simulink model "Lab2"  (R2024b)
settings: Solver=FixedStepAuto  StartTime=0.0  StopTime=10.0  RelTol=1e-3  EnableMultiTasking=on
undefined symbols (not defined in the file): BOOL, DINT, OTL, slplc
libraries: simulink x8, arduinolib x3
(part 2 of 8)

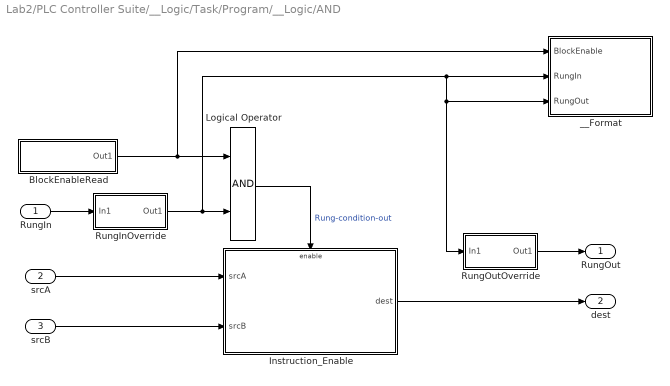
== system Lab2/PLC Controller Suite/__Logic/Task/Program/__Logic/AND ==
  RungIn : Inport  OutDataTypeStr=BOOL  PortDimensions=1
  srcA : Inport  Port=2  PortDimensions=1
  srcB : Inport  Port=3  PortDimensions=1
  BlockEnableRead : Subsystem  DisableCoverage=on  TreatAsAtomicUnit=on  mask{PLCLabelTag=_Block_Enable, PLCBlockType=BlockEnableRead}
      mask prompts: PLCLabelTag "Label Tag:"
      mask init:
      | block = gcb;
      | maskObj = Simulink.Mask.get(block);
      | maskObj.Display = sprintf('disp(''%s'');', PLCLabelTag);
      mask Help: web([docroot '/plccoder/ref/blockenableread' '.html']);
      mask DialogControl PLCBlockTitle Prompt: Block Enable Read
      mask Display: disp('_Block_Enable');
  Instruction_Enable : Subsystem  TreatAsAtomicUnit=on
  Logical Operator : Logic  OutDataTypeStr=BOOL
  RungInOverride : Subsystem  DisableCoverage=on  TreatAsAtomicUnit=on
  RungOutOverride : Subsystem  DisableCoverage=on  TreatAsAtomicUnit=on
  __Format : MATLAB Function  Tag=PLC_Format_FC  Priority=20  DisableCoverage=on  InitFcn=slplc.utils.setBlockAppearance('reset');  StopFcn=slplc.utils.setBlockAppearance('reset');  TreatAsAtomicUnit=on
  RungOut : Outport  OutDataTypeStr=BOOL  PortDimensions=1  VectorParamsAs1DForOutWhenUnconnected=off
  dest : Outport  Port=2  PortDimensions=1  VectorParamsAs1DForOutWhenUnconnected=off
  wires:
  RungOutOverride/1(Out1) -> RungOut/1
  RungIn/1 -> RungInOverride/1(In1)
  BlockEnableRead/1(Out1) -> Logical Operator/1, __Format/1(BlockEnable)
  srcB/1 -> Instruction_Enable/2(srcB)
  RungInOverride/1(Out1) -> Logical Operator/2, RungOutOverride/1(In1), __Format/3(RungOut), __Format/2(RungIn)
  Instruction_Enable/1(dest) -> dest/1
  srcA/1 -> Instruction_Enable/1(srcA)
  Logical Operator/1 -> Instruction_Enable/Enable  "Rung-condition-out"

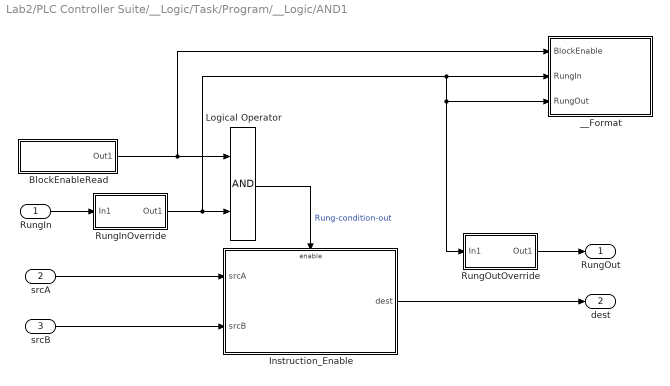
== system Lab2/PLC Controller Suite/__Logic/Task/Program/__Logic/AND1 ==
  RungIn : Inport  OutDataTypeStr=BOOL  PortDimensions=1
  srcA : Inport  Port=2  PortDimensions=1
  srcB : Inport  Port=3  PortDimensions=1
  BlockEnableRead : Subsystem  DisableCoverage=on  TreatAsAtomicUnit=on  mask{PLCLabelTag=_Block_Enable, PLCBlockType=BlockEnableRead}
      mask prompts: PLCLabelTag "Label Tag:"
      mask init:
      | block = gcb;
      | maskObj = Simulink.Mask.get(block);
      | maskObj.Display = sprintf('disp(''%s'');', PLCLabelTag);
      mask Help: web([docroot '/plccoder/ref/blockenableread' '.html']);
      mask DialogControl PLCBlockTitle Prompt: Block Enable Read
      mask Display: disp('_Block_Enable');
  Instruction_Enable : Subsystem  TreatAsAtomicUnit=on
  Logical Operator : Logic  OutDataTypeStr=BOOL
  RungInOverride : Subsystem  DisableCoverage=on  TreatAsAtomicUnit=on
  RungOutOverride : Subsystem  DisableCoverage=on  TreatAsAtomicUnit=on
  __Format : MATLAB Function  Tag=PLC_Format_FC  Priority=20  DisableCoverage=on  InitFcn=slplc.utils.setBlockAppearance('reset');  StopFcn=slplc.utils.setBlockAppearance('reset');  TreatAsAtomicUnit=on
  RungOut : Outport  OutDataTypeStr=BOOL  PortDimensions=1  VectorParamsAs1DForOutWhenUnconnected=off
  dest : Outport  Port=2  PortDimensions=1  VectorParamsAs1DForOutWhenUnconnected=off
  wires:
  RungOutOverride/1(Out1) -> RungOut/1
  RungIn/1 -> RungInOverride/1(In1)
  BlockEnableRead/1(Out1) -> Logical Operator/1, __Format/1(BlockEnable)
  srcB/1 -> Instruction_Enable/2(srcB)
  RungInOverride/1(Out1) -> Logical Operator/2, RungOutOverride/1(In1), __Format/3(RungOut), __Format/2(RungIn)
  Instruction_Enable/1(dest) -> dest/1
  srcA/1 -> Instruction_Enable/1(srcA)
  Logical Operator/1 -> Instruction_Enable/Enable  "Rung-condition-out"

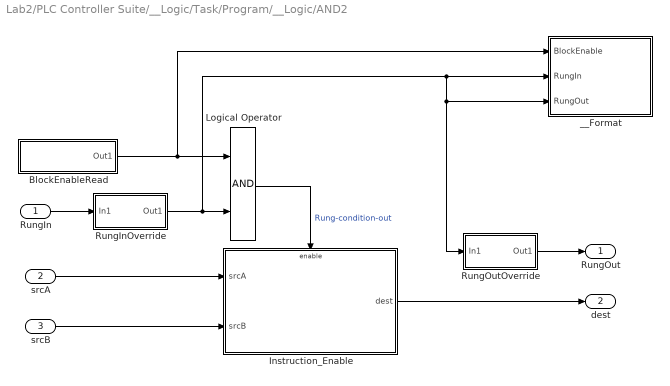
== system Lab2/PLC Controller Suite/__Logic/Task/Program/__Logic/AND2 ==
  RungIn : Inport  OutDataTypeStr=BOOL  PortDimensions=1
  srcA : Inport  Port=2  PortDimensions=1
  srcB : Inport  Port=3  PortDimensions=1
  BlockEnableRead : Subsystem  DisableCoverage=on  TreatAsAtomicUnit=on  mask{PLCLabelTag=_Block_Enable, PLCBlockType=BlockEnableRead}
      mask prompts: PLCLabelTag "Label Tag:"
      mask init:
      | block = gcb;
      | maskObj = Simulink.Mask.get(block);
      | maskObj.Display = sprintf('disp(''%s'');', PLCLabelTag);
      mask Help: web([docroot '/plccoder/ref/blockenableread' '.html']);
      mask DialogControl PLCBlockTitle Prompt: Block Enable Read
      mask Display: disp('_Block_Enable');
  Instruction_Enable : Subsystem  TreatAsAtomicUnit=on
  Logical Operator : Logic  OutDataTypeStr=BOOL
  RungInOverride : Subsystem  DisableCoverage=on  TreatAsAtomicUnit=on
  RungOutOverride : Subsystem  DisableCoverage=on  TreatAsAtomicUnit=on
  __Format : MATLAB Function  Tag=PLC_Format_FC  Priority=20  DisableCoverage=on  InitFcn=slplc.utils.setBlockAppearance('reset');  StopFcn=slplc.utils.setBlockAppearance('reset');  TreatAsAtomicUnit=on
  RungOut : Outport  OutDataTypeStr=BOOL  PortDimensions=1  VectorParamsAs1DForOutWhenUnconnected=off
  dest : Outport  Port=2  PortDimensions=1  VectorParamsAs1DForOutWhenUnconnected=off
  wires:
  RungOutOverride/1(Out1) -> RungOut/1
  RungIn/1 -> RungInOverride/1(In1)
  BlockEnableRead/1(Out1) -> Logical Operator/1, __Format/1(BlockEnable)
  srcB/1 -> Instruction_Enable/2(srcB)
  RungInOverride/1(Out1) -> Logical Operator/2, RungOutOverride/1(In1), __Format/3(RungOut), __Format/2(RungIn)
  Instruction_Enable/1(dest) -> dest/1
  srcA/1 -> Instruction_Enable/1(srcA)
  Logical Operator/1 -> Instruction_Enable/Enable  "Rung-condition-out"

== system Lab2/PLC Controller Suite/__Logic/Task/Program/__Logic/Add Rungs ==

== system Lab2/PLC Controller Suite/__Logic/Task/Program/__Logic/Add Single Rung ==

== system Lab2/PLC Controller Suite/__Logic/Task/Program/__Logic/Junction ==
  RungIn1 : Inport
  RungIn2 : Inport  Port=2
  BlockEnableRead : Subsystem  DisableCoverage=on  TreatAsAtomicUnit=on  mask{PLCLabelTag=_Block_Enable, PLCBlockType=BlockEnableRead}
      mask prompts: PLCLabelTag "Label Tag:"
      mask init:
      | block = gcb;
      | maskObj = Simulink.Mask.get(block);
      | maskObj.Display = sprintf('disp(''%s'');', PLCLabelTag);
      mask Help: web([docroot '/plccoder/ref/blockenableread' '.html']);
      mask DialogControl PLCBlockTitle Prompt: Block Enable Read
      mask Display: disp('_Block_Enable');
  __Enable : Subsystem  TreatAsAtomicUnit=on
  __Format : MATLAB Function  Tag=PLC_Format_Joint  Priority=20  DisableCoverage=on  InitFcn=slplc.utils.setBlockAppearance('reset', '', {'black', 'black'});  StopFcn=slplc.utils.setBlockAppearance('reset', '', {'black', 'black'});  TreatAsAtomicUnit=on
  RungOut : Outport  VectorParamsAs1DForOutWhenUnconnected=off
  wires:
  __Enable/1(RungOut) -> RungOut/1, __Format/2(RungOut)
  RungIn2/1 -> __Enable/2(RungIn2)
  RungIn1/1 -> __Enable/1(RungIn1)
  BlockEnableRead/1(Out1) -> __Enable/Enable, __Format/1(BlockEnable)

== system Lab2/PLC Controller Suite/__Logic/Task/Program/__Logic/Junction1 ==
  RungIn1 : Inport
  RungIn2 : Inport  Port=2
  BlockEnableRead : Subsystem  DisableCoverage=on  TreatAsAtomicUnit=on  mask{PLCLabelTag=_Block_Enable, PLCBlockType=BlockEnableRead}
      mask prompts: PLCLabelTag "Label Tag:"
      mask init:
      | block = gcb;
      | maskObj = Simulink.Mask.get(block);
      | maskObj.Display = sprintf('disp(''%s'');', PLCLabelTag);
      mask Help: web([docroot '/plccoder/ref/blockenableread' '.html']);
      mask DialogControl PLCBlockTitle Prompt: Block Enable Read
      mask Display: disp('_Block_Enable');
  __Enable : Subsystem  TreatAsAtomicUnit=on
  __Format : MATLAB Function  Tag=PLC_Format_Joint  Priority=20  DisableCoverage=on  InitFcn=slplc.utils.setBlockAppearance('reset', '', {'black', 'black'});  StopFcn=slplc.utils.setBlockAppearance('reset', '', {'black', 'black'});  TreatAsAtomicUnit=on
  RungOut : Outport  VectorParamsAs1DForOutWhenUnconnected=off
  wires:
  __Enable/1(RungOut) -> RungOut/1, __Format/2(RungOut)
  RungIn2/1 -> __Enable/2(RungIn2)
  RungIn1/1 -> __Enable/1(RungIn1)
  BlockEnableRead/1(Out1) -> __Enable/Enable, __Format/1(BlockEnable)

== system Lab2/PLC Controller Suite/__Logic/Task/Program/__Logic/Junction2 ==
  RungIn1 : Inport
  RungIn2 : Inport  Port=2
  BlockEnableRead : Subsystem  DisableCoverage=on  TreatAsAtomicUnit=on  mask{PLCLabelTag=_Block_Enable, PLCBlockType=BlockEnableRead}
      mask prompts: PLCLabelTag "Label Tag:"
      mask init:
      | block = gcb;
      | maskObj = Simulink.Mask.get(block);
      | maskObj.Display = sprintf('disp(''%s'');', PLCLabelTag);
      mask Help: web([docroot '/plccoder/ref/blockenableread' '.html']);
      mask DialogControl PLCBlockTitle Prompt: Block Enable Read
      mask Display: disp('_Block_Enable');
  __Enable : Subsystem  TreatAsAtomicUnit=on
  __Format : MATLAB Function  Tag=PLC_Format_Joint  Priority=20  DisableCoverage=on  InitFcn=slplc.utils.setBlockAppearance('reset', '', {'black', 'black'});  StopFcn=slplc.utils.setBlockAppearance('reset', '', {'black', 'black'});  TreatAsAtomicUnit=on
  RungOut : Outport  VectorParamsAs1DForOutWhenUnconnected=off
  wires:
  __Enable/1(RungOut) -> RungOut/1, __Format/2(RungOut)
  RungIn2/1 -> __Enable/2(RungIn2)
  RungIn1/1 -> __Enable/1(RungIn1)
  BlockEnableRead/1(Out1) -> __Enable/Enable, __Format/1(BlockEnable)

== system Lab2/PLC Controller Suite/__Logic/Task/Program/__Logic/Junction3 ==
  RungIn1 : Inport
  RungIn2 : Inport  Port=2
  BlockEnableRead : Subsystem  DisableCoverage=on  TreatAsAtomicUnit=on  mask{PLCLabelTag=_Block_Enable, PLCBlockType=BlockEnableRead}
      mask prompts: PLCLabelTag "Label Tag:"
      mask init:
      | block = gcb;
      | maskObj = Simulink.Mask.get(block);
      | maskObj.Display = sprintf('disp(''%s'');', PLCLabelTag);
      mask Help: web([docroot '/plccoder/ref/blockenableread' '.html']);
      mask DialogControl PLCBlockTitle Prompt: Block Enable Read
      mask Display: disp('_Block_Enable');
  __Enable : Subsystem  TreatAsAtomicUnit=on
  __Format : MATLAB Function  Tag=PLC_Format_Joint  Priority=20  DisableCoverage=on  InitFcn=slplc.utils.setBlockAppearance('reset', '', {'black', 'black'});  StopFcn=slplc.utils.setBlockAppearance('reset', '', {'black', 'black'});  TreatAsAtomicUnit=on
  RungOut : Outport  VectorParamsAs1DForOutWhenUnconnected=off
  wires:
  __Enable/1(RungOut) -> RungOut/1, __Format/2(RungOut)
  RungIn2/1 -> __Enable/2(RungIn2)
  RungIn1/1 -> __Enable/1(RungIn1)
  BlockEnableRead/1(Out1) -> __Enable/Enable, __Format/1(BlockEnable)

== system Lab2/PLC Controller Suite/__Logic/Task/Program/__Logic/Junction4 ==
  RungIn1 : Inport
  RungIn2 : Inport  Port=2
  BlockEnableRead : Subsystem  DisableCoverage=on  TreatAsAtomicUnit=on  mask{PLCLabelTag=_Block_Enable, PLCBlockType=BlockEnableRead}
      mask prompts: PLCLabelTag "Label Tag:"
      mask init:
      | block = gcb;
      | maskObj = Simulink.Mask.get(block);
      | maskObj.Display = sprintf('disp(''%s'');', PLCLabelTag);
      mask Help: web([docroot '/plccoder/ref/blockenableread' '.html']);
      mask DialogControl PLCBlockTitle Prompt: Block Enable Read
      mask Display: disp('_Block_Enable');
  __Enable : Subsystem  TreatAsAtomicUnit=on
  __Format : MATLAB Function  Tag=PLC_Format_Joint  Priority=20  DisableCoverage=on  InitFcn=slplc.utils.setBlockAppearance('reset', '', {'black', 'black'});  StopFcn=slplc.utils.setBlockAppearance('reset', '', {'black', 'black'});  TreatAsAtomicUnit=on
  RungOut : Outport  VectorParamsAs1DForOutWhenUnconnected=off
  wires:
  __Enable/1(RungOut) -> RungOut/1, __Format/2(RungOut)
  RungIn2/1 -> __Enable/2(RungIn2)
  RungIn1/1 -> __Enable/1(RungIn1)
  BlockEnableRead/1(Out1) -> __Enable/Enable, __Format/1(BlockEnable)

== system Lab2/PLC Controller Suite/__Logic/Task/Program/__Logic/LES ==
  RungIn : Inport  OutDataTypeStr=BOOL  PortDimensions=1
  srcA : Inport  Port=2  PortDimensions=1
  srcB : Inport  Port=3  PortDimensions=1
  BlockEnableRead : Subsystem  DisableCoverage=on  TreatAsAtomicUnit=on  mask{PLCLabelTag=_Block_Enable, PLCBlockType=BlockEnableRead}
      mask prompts: PLCLabelTag "Label Tag:"
      mask init:
      | block = gcb;
      | maskObj = Simulink.Mask.get(block);
      | maskObj.Display = sprintf('disp(''%s'');', PLCLabelTag);
      mask Help: web([docroot '/plccoder/ref/blockenableread' '.html']);
      mask DialogControl PLCBlockTitle Prompt: Block Enable Read
      mask Display: disp('_Block_Enable');
  Instruction_Enable : Subsystem  TreatAsAtomicUnit=on
  RungInOverride : Subsystem  DisableCoverage=on  TreatAsAtomicUnit=on
  __Format : MATLAB Function  Tag=PLC_Format_FC  Priority=20  DisableCoverage=on  InitFcn=slplc.utils.setBlockAppearance('reset');  StopFcn=slplc.utils.setBlockAppearance('reset');  TreatAsAtomicUnit=on
  RungOut : Outport  OutDataTypeStr=BOOL  PortDimensions=1  VectorParamsAs1DForOutWhenUnconnected=off
  wires:
  RungIn/1 -> RungInOverride/1(In1)
  srcB/1 -> Instruction_Enable/3(srcB)
  Instruction_Enable/1(Rung-condition-out) -> RungOut/1, __Format/3(RungOut)
  BlockEnableRead/1(Out1) -> Instruction_Enable/Enable, __Format/1(BlockEnable)
  RungInOverride/1(Out1) -> Instruction_Enable/1(Rung-condition-in), __Format/2(RungIn)
  srcA/1 -> Instruction_Enable/2(srcA)

== system Lab2/PLC Controller Suite/__Logic/Task/Program/__Logic/LES1 ==
  RungIn : Inport  OutDataTypeStr=BOOL  PortDimensions=1
  srcA : Inport  Port=2  PortDimensions=1
  srcB : Inport  Port=3  PortDimensions=1
  BlockEnableRead : Subsystem  DisableCoverage=on  TreatAsAtomicUnit=on  mask{PLCLabelTag=_Block_Enable, PLCBlockType=BlockEnableRead}
      mask prompts: PLCLabelTag "Label Tag:"
      mask init:
      | block = gcb;
      | maskObj = Simulink.Mask.get(block);
      | maskObj.Display = sprintf('disp(''%s'');', PLCLabelTag);
      mask Help: web([docroot '/plccoder/ref/blockenableread' '.html']);
      mask DialogControl PLCBlockTitle Prompt: Block Enable Read
      mask Display: disp('_Block_Enable');
  Instruction_Enable : Subsystem  TreatAsAtomicUnit=on
  RungInOverride : Subsystem  DisableCoverage=on  TreatAsAtomicUnit=on
  __Format : MATLAB Function  Tag=PLC_Format_FC  Priority=20  DisableCoverage=on  InitFcn=slplc.utils.setBlockAppearance('reset');  StopFcn=slplc.utils.setBlockAppearance('reset');  TreatAsAtomicUnit=on
  RungOut : Outport  OutDataTypeStr=BOOL  PortDimensions=1  VectorParamsAs1DForOutWhenUnconnected=off
  wires:
  RungIn/1 -> RungInOverride/1(In1)
  srcB/1 -> Instruction_Enable/3(srcB)
  Instruction_Enable/1(Rung-condition-out) -> RungOut/1, __Format/3(RungOut)
  BlockEnableRead/1(Out1) -> Instruction_Enable/Enable, __Format/1(BlockEnable)
  RungInOverride/1(Out1) -> Instruction_Enable/1(Rung-condition-in), __Format/2(RungIn)
  srcA/1 -> Instruction_Enable/2(srcA)

== system Lab2/PLC Controller Suite/__Logic/Task/Program/__Logic/LES2 ==
  RungIn : Inport  OutDataTypeStr=BOOL  PortDimensions=1
  srcA : Inport  Port=2  PortDimensions=1
  srcB : Inport  Port=3  PortDimensions=1
  BlockEnableRead : Subsystem  DisableCoverage=on  TreatAsAtomicUnit=on  mask{PLCLabelTag=_Block_Enable, PLCBlockType=BlockEnableRead}
      mask prompts: PLCLabelTag "Label Tag:"
      mask init:
      | block = gcb;
      | maskObj = Simulink.Mask.get(block);
      | maskObj.Display = sprintf('disp(''%s'');', PLCLabelTag);
      mask Help: web([docroot '/plccoder/ref/blockenableread' '.html']);
      mask DialogControl PLCBlockTitle Prompt: Block Enable Read
      mask Display: disp('_Block_Enable');
  Instruction_Enable : Subsystem  TreatAsAtomicUnit=on
  RungInOverride : Subsystem  DisableCoverage=on  TreatAsAtomicUnit=on
  __Format : MATLAB Function  Tag=PLC_Format_FC  Priority=20  DisableCoverage=on  InitFcn=slplc.utils.setBlockAppearance('reset');  StopFcn=slplc.utils.setBlockAppearance('reset');  TreatAsAtomicUnit=on
  RungOut : Outport  OutDataTypeStr=BOOL  PortDimensions=1  VectorParamsAs1DForOutWhenUnconnected=off
  wires:
  RungIn/1 -> RungInOverride/1(In1)
  srcB/1 -> Instruction_Enable/3(srcB)
  Instruction_Enable/1(Rung-condition-out) -> RungOut/1, __Format/3(RungOut)
  BlockEnableRead/1(Out1) -> Instruction_Enable/Enable, __Format/1(BlockEnable)
  RungInOverride/1(Out1) -> Instruction_Enable/1(Rung-condition-in), __Format/2(RungIn)
  srcA/1 -> Instruction_Enable/2(srcA)

== system Lab2/PLC Controller Suite/__Logic/Task/Program/__Logic/LES3 ==
  RungIn : Inport  OutDataTypeStr=BOOL  PortDimensions=1
  srcA : Inport  Port=2  PortDimensions=1
  srcB : Inport  Port=3  PortDimensions=1
  BlockEnableRead : Subsystem  DisableCoverage=on  TreatAsAtomicUnit=on  mask{PLCLabelTag=_Block_Enable, PLCBlockType=BlockEnableRead}
      mask prompts: PLCLabelTag "Label Tag:"
      mask init:
      | block = gcb;
      | maskObj = Simulink.Mask.get(block);
      | maskObj.Display = sprintf('disp(''%s'');', PLCLabelTag);
      mask Help: web([docroot '/plccoder/ref/blockenableread' '.html']);
      mask DialogControl PLCBlockTitle Prompt: Block Enable Read
      mask Display: disp('_Block_Enable');
  Instruction_Enable : Subsystem  TreatAsAtomicUnit=on
  RungInOverride : Subsystem  DisableCoverage=on  TreatAsAtomicUnit=on
  __Format : MATLAB Function  Tag=PLC_Format_FC  Priority=20  DisableCoverage=on  InitFcn=slplc.utils.setBlockAppearance('reset');  StopFcn=slplc.utils.setBlockAppearance('reset');  TreatAsAtomicUnit=on
  RungOut : Outport  OutDataTypeStr=BOOL  PortDimensions=1  VectorParamsAs1DForOutWhenUnconnected=off
  wires:
  RungIn/1 -> RungInOverride/1(In1)
  srcB/1 -> Instruction_Enable/3(srcB)
  Instruction_Enable/1(Rung-condition-out) -> RungOut/1, __Format/3(RungOut)
  BlockEnableRead/1(Out1) -> Instruction_Enable/Enable, __Format/1(BlockEnable)
  RungInOverride/1(Out1) -> Instruction_Enable/1(Rung-condition-in), __Format/2(RungIn)
  srcA/1 -> Instruction_Enable/2(srcA)

== system Lab2/PLC Controller Suite/__Logic/Task/Program/__Logic/LES4 ==
  RungIn : Inport  OutDataTypeStr=BOOL  PortDimensions=1
  srcA : Inport  Port=2  PortDimensions=1
  srcB : Inport  Port=3  PortDimensions=1
  BlockEnableRead : Subsystem  DisableCoverage=on  TreatAsAtomicUnit=on  mask{PLCLabelTag=_Block_Enable, PLCBlockType=BlockEnableRead}
      mask prompts: PLCLabelTag "Label Tag:"
      mask init:
      | block = gcb;
      | maskObj = Simulink.Mask.get(block);
      | maskObj.Display = sprintf('disp(''%s'');', PLCLabelTag);
      mask Help: web([docroot '/plccoder/ref/blockenableread' '.html']);
      mask DialogControl PLCBlockTitle Prompt: Block Enable Read
      mask Display: disp('_Block_Enable');
  Instruction_Enable : Subsystem  TreatAsAtomicUnit=on
  RungInOverride : Subsystem  DisableCoverage=on  TreatAsAtomicUnit=on
  __Format : MATLAB Function  Tag=PLC_Format_FC  Priority=20  DisableCoverage=on  InitFcn=slplc.utils.setBlockAppearance('reset');  StopFcn=slplc.utils.setBlockAppearance('reset');  TreatAsAtomicUnit=on
  RungOut : Outport  OutDataTypeStr=BOOL  PortDimensions=1  VectorParamsAs1DForOutWhenUnconnected=off
  wires:
  RungIn/1 -> RungInOverride/1(In1)
  srcB/1 -> Instruction_Enable/3(srcB)
  Instruction_Enable/1(Rung-condition-out) -> RungOut/1, __Format/3(RungOut)
  BlockEnableRead/1(Out1) -> Instruction_Enable/Enable, __Format/1(BlockEnable)
  RungInOverride/1(Out1) -> Instruction_Enable/1(Rung-condition-in), __Format/2(RungIn)
  srcA/1 -> Instruction_Enable/2(srcA)

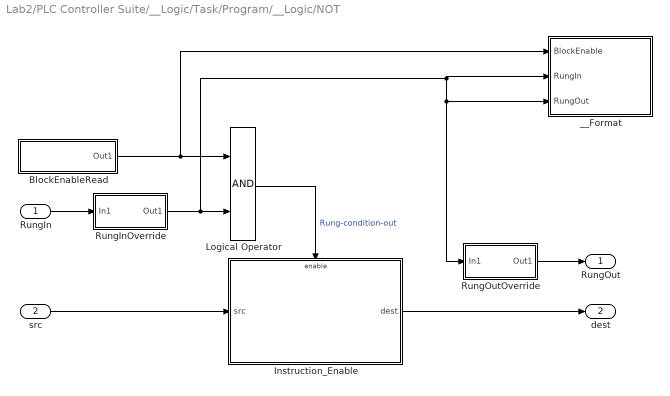
== system Lab2/PLC Controller Suite/__Logic/Task/Program/__Logic/NOT ==
  RungIn : Inport  OutDataTypeStr=BOOL  PortDimensions=1
  src : Inport  Port=2  PortDimensions=1
  BlockEnableRead : Subsystem  DisableCoverage=on  TreatAsAtomicUnit=on  mask{PLCLabelTag=_Block_Enable, PLCBlockType=BlockEnableRead}
      mask prompts: PLCLabelTag "Label Tag:"
      mask init:
      | block = gcb;
      | maskObj = Simulink.Mask.get(block);
      | maskObj.Display = sprintf('disp(''%s'');', PLCLabelTag);
      mask Help: web([docroot '/plccoder/ref/blockenableread' '.html']);
      mask DialogControl PLCBlockTitle Prompt: Block Enable Read
      mask Display: disp('_Block_Enable');
  Instruction_Enable : Subsystem  TreatAsAtomicUnit=on
  Logical Operator : Logic  OutDataTypeStr=BOOL
  RungInOverride : Subsystem  DisableCoverage=on  TreatAsAtomicUnit=on
  RungOutOverride : Subsystem  DisableCoverage=on  TreatAsAtomicUnit=on
  __Format : MATLAB Function  Tag=PLC_Format_FC  Priority=20  DisableCoverage=on  InitFcn=slplc.utils.setBlockAppearance('reset');  StopFcn=slplc.utils.setBlockAppearance('reset');  TreatAsAtomicUnit=on
  RungOut : Outport  OutDataTypeStr=BOOL  PortDimensions=1  VectorParamsAs1DForOutWhenUnconnected=off
  dest : Outport  Port=2  PortDimensions=1  VectorParamsAs1DForOutWhenUnconnected=off
  wires:
  BlockEnableRead/1(Out1) -> Logical Operator/1, __Format/1(BlockEnable)
  RungInOverride/1(Out1) -> RungOutOverride/1(In1), __Format/3(RungOut), __Format/2(RungIn), Logical Operator/2
  RungOutOverride/1(Out1) -> RungOut/1
  src/1 -> Instruction_Enable/1(src)
  RungIn/1 -> RungInOverride/1(In1)
  Instruction_Enable/1(dest) -> dest/1
  Logical Operator/1 -> Instruction_Enable/Enable  "Rung-condition-out"

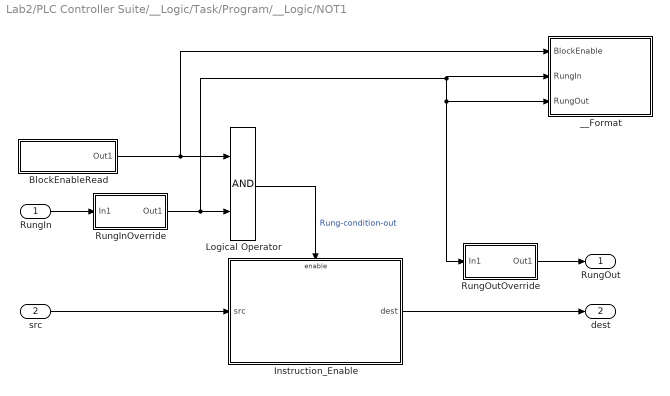
== system Lab2/PLC Controller Suite/__Logic/Task/Program/__Logic/NOT1 ==
  RungIn : Inport  OutDataTypeStr=BOOL  PortDimensions=1
  src : Inport  Port=2  PortDimensions=1
  BlockEnableRead : Subsystem  DisableCoverage=on  TreatAsAtomicUnit=on  mask{PLCLabelTag=_Block_Enable, PLCBlockType=BlockEnableRead}
      mask prompts: PLCLabelTag "Label Tag:"
      mask init:
      | block = gcb;
      | maskObj = Simulink.Mask.get(block);
      | maskObj.Display = sprintf('disp(''%s'');', PLCLabelTag);
      mask Help: web([docroot '/plccoder/ref/blockenableread' '.html']);
      mask DialogControl PLCBlockTitle Prompt: Block Enable Read
      mask Display: disp('_Block_Enable');
  Instruction_Enable : Subsystem  TreatAsAtomicUnit=on
  Logical Operator : Logic  OutDataTypeStr=BOOL
  RungInOverride : Subsystem  DisableCoverage=on  TreatAsAtomicUnit=on
  RungOutOverride : Subsystem  DisableCoverage=on  TreatAsAtomicUnit=on
  __Format : MATLAB Function  Tag=PLC_Format_FC  Priority=20  DisableCoverage=on  InitFcn=slplc.utils.setBlockAppearance('reset');  StopFcn=slplc.utils.setBlockAppearance('reset');  TreatAsAtomicUnit=on
  RungOut : Outport  OutDataTypeStr=BOOL  PortDimensions=1  VectorParamsAs1DForOutWhenUnconnected=off
  dest : Outport  Port=2  PortDimensions=1  VectorParamsAs1DForOutWhenUnconnected=off
  wires:
  BlockEnableRead/1(Out1) -> Logical Operator/1, __Format/1(BlockEnable)
  RungInOverride/1(Out1) -> RungOutOverride/1(In1), __Format/3(RungOut), __Format/2(RungIn), Logical Operator/2
  RungOutOverride/1(Out1) -> RungOut/1
  src/1 -> Instruction_Enable/1(src)
  RungIn/1 -> RungInOverride/1(In1)
  Instruction_Enable/1(dest) -> dest/1
  Logical Operator/1 -> Instruction_Enable/Enable  "Rung-condition-out"

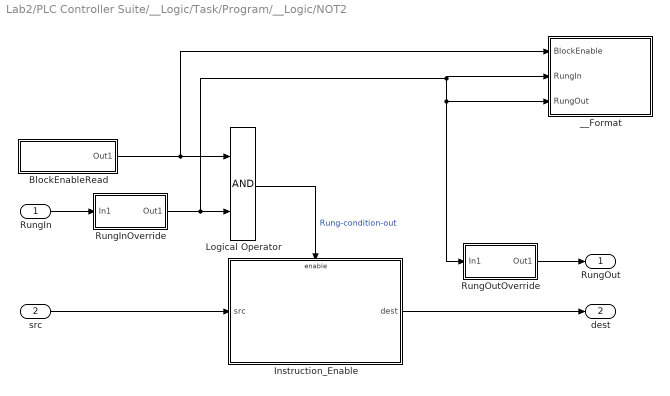
== system Lab2/PLC Controller Suite/__Logic/Task/Program/__Logic/NOT2 ==
  RungIn : Inport  OutDataTypeStr=BOOL  PortDimensions=1
  src : Inport  Port=2  PortDimensions=1
  BlockEnableRead : Subsystem  DisableCoverage=on  TreatAsAtomicUnit=on  mask{PLCLabelTag=_Block_Enable, PLCBlockType=BlockEnableRead}
      mask prompts: PLCLabelTag "Label Tag:"
      mask init:
      | block = gcb;
      | maskObj = Simulink.Mask.get(block);
      | maskObj.Display = sprintf('disp(''%s'');', PLCLabelTag);
      mask Help: web([docroot '/plccoder/ref/blockenableread' '.html']);
      mask DialogControl PLCBlockTitle Prompt: Block Enable Read
      mask Display: disp('_Block_Enable');
  Instruction_Enable : Subsystem  TreatAsAtomicUnit=on
  Logical Operator : Logic  OutDataTypeStr=BOOL
  RungInOverride : Subsystem  DisableCoverage=on  TreatAsAtomicUnit=on
  RungOutOverride : Subsystem  DisableCoverage=on  TreatAsAtomicUnit=on
  __Format : MATLAB Function  Tag=PLC_Format_FC  Priority=20  DisableCoverage=on  InitFcn=slplc.utils.setBlockAppearance('reset');  StopFcn=slplc.utils.setBlockAppearance('reset');  TreatAsAtomicUnit=on
  RungOut : Outport  OutDataTypeStr=BOOL  PortDimensions=1  VectorParamsAs1DForOutWhenUnconnected=off
  dest : Outport  Port=2  PortDimensions=1  VectorParamsAs1DForOutWhenUnconnected=off
  wires:
  BlockEnableRead/1(Out1) -> Logical Operator/1, __Format/1(BlockEnable)
  RungInOverride/1(Out1) -> RungOutOverride/1(In1), __Format/3(RungOut), __Format/2(RungIn), Logical Operator/2
  RungOutOverride/1(Out1) -> RungOut/1
  src/1 -> Instruction_Enable/1(src)
  RungIn/1 -> RungInOverride/1(In1)
  Instruction_Enable/1(dest) -> dest/1
  Logical Operator/1 -> Instruction_Enable/Enable  "Rung-condition-out"

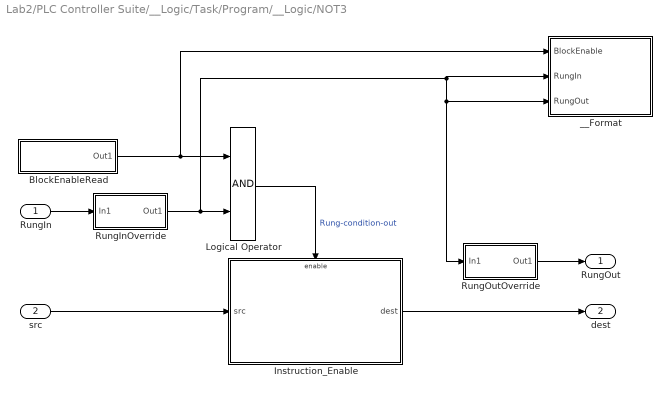
== system Lab2/PLC Controller Suite/__Logic/Task/Program/__Logic/NOT3 ==
  RungIn : Inport  OutDataTypeStr=BOOL  PortDimensions=1
  src : Inport  Port=2  PortDimensions=1
  BlockEnableRead : Subsystem  DisableCoverage=on  TreatAsAtomicUnit=on  mask{PLCLabelTag=_Block_Enable, PLCBlockType=BlockEnableRead}
      mask prompts: PLCLabelTag "Label Tag:"
      mask init:
      | block = gcb;
      | maskObj = Simulink.Mask.get(block);
      | maskObj.Display = sprintf('disp(''%s'');', PLCLabelTag);
      mask Help: web([docroot '/plccoder/ref/blockenableread' '.html']);
      mask DialogControl PLCBlockTitle Prompt: Block Enable Read
      mask Display: disp('_Block_Enable');
  Instruction_Enable : Subsystem  TreatAsAtomicUnit=on
  Logical Operator : Logic  OutDataTypeStr=BOOL
  RungInOverride : Subsystem  DisableCoverage=on  TreatAsAtomicUnit=on
  RungOutOverride : Subsystem  DisableCoverage=on  TreatAsAtomicUnit=on
  __Format : MATLAB Function  Tag=PLC_Format_FC  Priority=20  DisableCoverage=on  InitFcn=slplc.utils.setBlockAppearance('reset');  StopFcn=slplc.utils.setBlockAppearance('reset');  TreatAsAtomicUnit=on
  RungOut : Outport  OutDataTypeStr=BOOL  PortDimensions=1  VectorParamsAs1DForOutWhenUnconnected=off
  dest : Outport  Port=2  PortDimensions=1  VectorParamsAs1DForOutWhenUnconnected=off
  wires:
  BlockEnableRead/1(Out1) -> Logical Operator/1, __Format/1(BlockEnable)
  RungInOverride/1(Out1) -> RungOutOverride/1(In1), __Format/3(RungOut), __Format/2(RungIn), Logical Operator/2
  RungOutOverride/1(Out1) -> RungOut/1
  src/1 -> Instruction_Enable/1(src)
  RungIn/1 -> RungInOverride/1(In1)
  Instruction_Enable/1(dest) -> dest/1
  Logical Operator/1 -> Instruction_Enable/Enable  "Rung-condition-out"

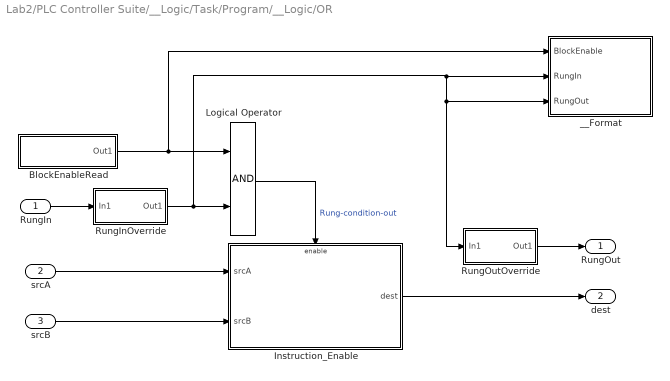
== system Lab2/PLC Controller Suite/__Logic/Task/Program/__Logic/OR ==
  RungIn : Inport  OutDataTypeStr=BOOL  PortDimensions=1
  srcA : Inport  Port=2  PortDimensions=1
  srcB : Inport  Port=3  PortDimensions=1
  BlockEnableRead : Subsystem  DisableCoverage=on  TreatAsAtomicUnit=on  mask{PLCLabelTag=_Block_Enable, PLCBlockType=BlockEnableRead}
      mask prompts: PLCLabelTag "Label Tag:"
      mask init:
      | block = gcb;
      | maskObj = Simulink.Mask.get(block);
      | maskObj.Display = sprintf('disp(''%s'');', PLCLabelTag);
      mask Help: web([docroot '/plccoder/ref/blockenableread' '.html']);
      mask DialogControl PLCBlockTitle Prompt: Block Enable Read
      mask Display: disp('_Block_Enable');
  Instruction_Enable : Subsystem  TreatAsAtomicUnit=on
  Logical Operator : Logic  OutDataTypeStr=BOOL
  RungInOverride : Subsystem  DisableCoverage=on  TreatAsAtomicUnit=on
  RungOutOverride : Subsystem  DisableCoverage=on  TreatAsAtomicUnit=on
  __Format : MATLAB Function  Tag=PLC_Format_FC  Priority=20  DisableCoverage=on  InitFcn=slplc.utils.setBlockAppearance('reset');  StopFcn=slplc.utils.setBlockAppearance('reset');  TreatAsAtomicUnit=on
  RungOut : Outport  OutDataTypeStr=BOOL  PortDimensions=1  VectorParamsAs1DForOutWhenUnconnected=off
  dest : Outport  Port=2  PortDimensions=1  VectorParamsAs1DForOutWhenUnconnected=off
  wires:
  RungIn/1 -> RungInOverride/1(In1)
  RungInOverride/1(Out1) -> RungOutOverride/1(In1), __Format/3(RungOut), __Format/2(RungIn), Logical Operator/2
  srcA/1 -> Instruction_Enable/1(srcA)
  Instruction_Enable/1(dest) -> dest/1
  BlockEnableRead/1(Out1) -> Logical Operator/1, __Format/1(BlockEnable)
  srcB/1 -> Instruction_Enable/2(srcB)
  RungOutOverride/1(Out1) -> RungOut/1
  Logical Operator/1 -> Instruction_Enable/Enable  "Rung-condition-out"

== system Lab2/PLC Controller Suite/__Logic/Task/Program/__Logic/OTE ==
  RungIn : Inport  PortDimensions=1
  BlockEnableRead : Subsystem  DisableCoverage=on  TreatAsAtomicUnit=on  mask{PLCLabelTag=_Block_Enable, PLCBlockType=BlockEnableRead}
      mask prompts: PLCLabelTag "Label Tag:"
      mask init:
      | block = gcb;
      | maskObj = Simulink.Mask.get(block);
      | maskObj.Display = sprintf('disp(''%s'');', PLCLabelTag);
      mask Help: web([docroot '/plccoder/ref/blockenableread' '.html']);
      mask DialogControl PLCBlockTitle Prompt: Block Enable Read
      mask Display: disp('_Block_Enable');
  Instruction_Enable : Subsystem  Priority=12  TreatAsAtomicUnit=on
  RungInOverride : Subsystem  DisableCoverage=on  TreatAsAtomicUnit=on
  __CoreVarRead : Subsystem  Tag=CoreVarReadBlock  DisableCoverage=on  TreatAsAtomicUnit=on  mask{PLCBlockType=CoreVarRead}
      mask init:
      | slplc.callbacks.initCoreVariable(gcb, 'read');
      mask Help: web([docroot '/plccoder/ref/__corevarread' '.html']);
      mask DialogControl PLCBlockTitle Prompt: Core Variable Read
  __Format : MATLAB Function  Tag=PLC_Format_Boolean  Priority=20  DisableCoverage=on  InitFcn=slplc.utils.setBlockAppearance('reset', '%<PLCOperandTag>');  StopFcn=slplc.utils.setBlockAppearance('reset', '%<PLCOperandTag>');  TreatAsAtomicUnit=on
  RungOut : Outport  OutDataTypeStr=BOOL  PortDimensions=1  InitialOutput=false  VectorParamsAs1DForOutWhenUnconnected=off
  wires:
  RungIn/1 -> RungInOverride/1(In1)
  BlockEnableRead/1(Out1) -> __Format/1(BlockEnable), Instruction_Enable/Enable
  RungInOverride/1(Out1) -> __Format/2(RungIn), __Format/3(RungOut), RungOut/1, Instruction_Enable/1(Rung-condition-in)
  __CoreVarRead/1(y) -> __Format/4(data)

== system Lab2/PLC Controller Suite/__Logic/Task/Program/__Logic/OTE1 ==
  RungIn : Inport  PortDimensions=1
  BlockEnableRead : Subsystem  DisableCoverage=on  TreatAsAtomicUnit=on  mask{PLCLabelTag=_Block_Enable, PLCBlockType=BlockEnableRead}
      mask prompts: PLCLabelTag "Label Tag:"
      mask init:
      | block = gcb;
      | maskObj = Simulink.Mask.get(block);
      | maskObj.Display = sprintf('disp(''%s'');', PLCLabelTag);
      mask Help: web([docroot '/plccoder/ref/blockenableread' '.html']);
      mask DialogControl PLCBlockTitle Prompt: Block Enable Read
      mask Display: disp('_Block_Enable');
  Instruction_Enable : Subsystem  Priority=12  TreatAsAtomicUnit=on
  RungInOverride : Subsystem  DisableCoverage=on  TreatAsAtomicUnit=on
  __CoreVarRead : Subsystem  Tag=CoreVarReadBlock  DisableCoverage=on  TreatAsAtomicUnit=on  mask{PLCBlockType=CoreVarRead}
      mask init:
      | slplc.callbacks.initCoreVariable(gcb, 'read');
      mask Help: web([docroot '/plccoder/ref/__corevarread' '.html']);
      mask DialogControl PLCBlockTitle Prompt: Core Variable Read
  __Format : MATLAB Function  Tag=PLC_Format_Boolean  Priority=20  DisableCoverage=on  InitFcn=slplc.utils.setBlockAppearance('reset', '%<PLCOperandTag>');  StopFcn=slplc.utils.setBlockAppearance('reset', '%<PLCOperandTag>');  TreatAsAtomicUnit=on
  RungOut : Outport  OutDataTypeStr=BOOL  PortDimensions=1  InitialOutput=false  VectorParamsAs1DForOutWhenUnconnected=off
  wires:
  RungIn/1 -> RungInOverride/1(In1)
  BlockEnableRead/1(Out1) -> __Format/1(BlockEnable), Instruction_Enable/Enable
  RungInOverride/1(Out1) -> __Format/2(RungIn), __Format/3(RungOut), RungOut/1, Instruction_Enable/1(Rung-condition-in)
  __CoreVarRead/1(y) -> __Format/4(data)

== system Lab2/PLC Controller Suite/__Logic/Task/Program/__Logic/OTE2 ==
  RungIn : Inport  PortDimensions=1
  BlockEnableRead : Subsystem  DisableCoverage=on  TreatAsAtomicUnit=on  mask{PLCLabelTag=_Block_Enable, PLCBlockType=BlockEnableRead}
      mask prompts: PLCLabelTag "Label Tag:"
      mask init:
      | block = gcb;
      | maskObj = Simulink.Mask.get(block);
      | maskObj.Display = sprintf('disp(''%s'');', PLCLabelTag);
      mask Help: web([docroot '/plccoder/ref/blockenableread' '.html']);
      mask DialogControl PLCBlockTitle Prompt: Block Enable Read
      mask Display: disp('_Block_Enable');
  Instruction_Enable : Subsystem  Priority=12  TreatAsAtomicUnit=on
  RungInOverride : Subsystem  DisableCoverage=on  TreatAsAtomicUnit=on
  __CoreVarRead : Subsystem  Tag=CoreVarReadBlock  DisableCoverage=on  TreatAsAtomicUnit=on  mask{PLCBlockType=CoreVarRead}
      mask init:
      | slplc.callbacks.initCoreVariable(gcb, 'read');
      mask Help: web([docroot '/plccoder/ref/__corevarread' '.html']);
      mask DialogControl PLCBlockTitle Prompt: Core Variable Read
  __Format : MATLAB Function  Tag=PLC_Format_Boolean  Priority=20  DisableCoverage=on  InitFcn=slplc.utils.setBlockAppearance('reset', '%<PLCOperandTag>');  StopFcn=slplc.utils.setBlockAppearance('reset', '%<PLCOperandTag>');  TreatAsAtomicUnit=on
  RungOut : Outport  OutDataTypeStr=BOOL  PortDimensions=1  InitialOutput=false  VectorParamsAs1DForOutWhenUnconnected=off
  wires:
  RungIn/1 -> RungInOverride/1(In1)
  BlockEnableRead/1(Out1) -> __Format/1(BlockEnable), Instruction_Enable/Enable
  RungInOverride/1(Out1) -> __Format/2(RungIn), __Format/3(RungOut), RungOut/1, Instruction_Enable/1(Rung-condition-in)
  __CoreVarRead/1(y) -> __Format/4(data)

== system Lab2/PLC Controller Suite/__Logic/Task/Program/__Logic/OTE3 ==
  RungIn : Inport  PortDimensions=1
  BlockEnableRead : Subsystem  DisableCoverage=on  TreatAsAtomicUnit=on  mask{PLCLabelTag=_Block_Enable, PLCBlockType=BlockEnableRead}
      mask prompts: PLCLabelTag "Label Tag:"
      mask init:
      | block = gcb;
      | maskObj = Simulink.Mask.get(block);
      | maskObj.Display = sprintf('disp(''%s'');', PLCLabelTag);
      mask Help: web([docroot '/plccoder/ref/blockenableread' '.html']);
      mask DialogControl PLCBlockTitle Prompt: Block Enable Read
      mask Display: disp('_Block_Enable');
  Instruction_Enable : Subsystem  Priority=12  TreatAsAtomicUnit=on
  RungInOverride : Subsystem  DisableCoverage=on  TreatAsAtomicUnit=on
  __CoreVarRead : Subsystem  Tag=CoreVarReadBlock  DisableCoverage=on  TreatAsAtomicUnit=on  mask{PLCBlockType=CoreVarRead}
      mask init:
      | slplc.callbacks.initCoreVariable(gcb, 'read');
      mask Help: web([docroot '/plccoder/ref/__corevarread' '.html']);
      mask DialogControl PLCBlockTitle Prompt: Core Variable Read
  __Format : MATLAB Function  Tag=PLC_Format_Boolean  Priority=20  DisableCoverage=on  InitFcn=slplc.utils.setBlockAppearance('reset', '%<PLCOperandTag>');  StopFcn=slplc.utils.setBlockAppearance('reset', '%<PLCOperandTag>');  TreatAsAtomicUnit=on
  RungOut : Outport  OutDataTypeStr=BOOL  PortDimensions=1  InitialOutput=false  VectorParamsAs1DForOutWhenUnconnected=off
  wires:
  RungIn/1 -> RungInOverride/1(In1)
  BlockEnableRead/1(Out1) -> __Format/1(BlockEnable), Instruction_Enable/Enable
  RungInOverride/1(Out1) -> __Format/2(RungIn), __Format/3(RungOut), RungOut/1, Instruction_Enable/1(Rung-condition-in)
  __CoreVarRead/1(y) -> __Format/4(data)

== system Lab2/PLC Controller Suite/__Logic/Task/Program/__Logic/OTL ==
  RungIn : Inport  PortDimensions=1
  BlockEnableRead : Subsystem  DisableCoverage=on  TreatAsAtomicUnit=on  mask{PLCLabelTag=_Block_Enable, PLCBlockType=BlockEnableRead}
      mask prompts: PLCLabelTag "Label Tag:"
      mask init:
      | block = gcb;
      | maskObj = Simulink.Mask.get(block);
      | maskObj.Display = sprintf('disp(''%s'');', PLCLabelTag);
      mask Help: web([docroot '/plccoder/ref/blockenableread' '.html']);
      mask DialogControl PLCBlockTitle Prompt: Block Enable Read
      mask Display: disp('_Block_Enable');
  Instruction_Enable : Subsystem  Priority=12  TreatAsAtomicUnit=on
  RungInOverride : Subsystem  DisableCoverage=on  TreatAsAtomicUnit=on
  __CoreVarRead : Subsystem  Tag=CoreVarReadBlock  DisableCoverage=on  TreatAsAtomicUnit=on  mask{PLCBlockType=CoreVarRead}
      mask init:
      | slplc.callbacks.initCoreVariable(gcb, 'read');
      mask Help: web([docroot '/plccoder/ref/__corevarread' '.html']);
      mask DialogControl PLCBlockTitle Prompt: Core Variable Read
  __Format : MATLAB Function  Tag=PLC_Format_Boolean  Priority=20  DisableCoverage=on  InitFcn=slplc.utils.setBlockAppearance('reset', '%<PLCOperandTag>');  StopFcn=slplc.utils.setBlockAppearance('reset', '%<PLCOperandTag>');  TreatAsAtomicUnit=on
  RungOut : Outport  OutDataTypeStr=BOOL  PortDimensions=1  InitialOutput=false  VectorParamsAs1DForOutWhenUnconnected=off
  wires:
  BlockEnableRead/1(Out1) -> Instruction_Enable/Enable, __Format/1(BlockEnable)
  RungIn/1 -> RungInOverride/1(In1)
  RungInOverride/1(Out1) -> Instruction_Enable/1(Rung-condition-in), __Format/3(RungOut), __Format/2(RungIn), RungOut/1
  __CoreVarRead/1(y) -> __Format/4(data)

== system Lab2/PLC Controller Suite/__Logic/Task/Program/__Logic/OTL1 ==
  RungIn : Inport  PortDimensions=1
  BlockEnableRead : Subsystem  DisableCoverage=on  TreatAsAtomicUnit=on  mask{PLCLabelTag=_Block_Enable, PLCBlockType=BlockEnableRead}
      mask prompts: PLCLabelTag "Label Tag:"
      mask init:
      | block = gcb;
      | maskObj = Simulink.Mask.get(block);
      | maskObj.Display = sprintf('disp(''%s'');', PLCLabelTag);
      mask Help: web([docroot '/plccoder/ref/blockenableread' '.html']);
      mask DialogControl PLCBlockTitle Prompt: Block Enable Read
      mask Display: disp('_Block_Enable');
  Instruction_Enable : Subsystem  Priority=12  TreatAsAtomicUnit=on
  RungInOverride : Subsystem  DisableCoverage=on  TreatAsAtomicUnit=on
  __CoreVarRead : Subsystem  Tag=CoreVarReadBlock  DisableCoverage=on  TreatAsAtomicUnit=on  mask{PLCBlockType=CoreVarRead}
      mask init:
      | slplc.callbacks.initCoreVariable(gcb, 'read');
      mask Help: web([docroot '/plccoder/ref/__corevarread' '.html']);
      mask DialogControl PLCBlockTitle Prompt: Core Variable Read
  __Format : MATLAB Function  Tag=PLC_Format_Boolean  Priority=20  DisableCoverage=on  InitFcn=slplc.utils.setBlockAppearance('reset', '%<PLCOperandTag>');  StopFcn=slplc.utils.setBlockAppearance('reset', '%<PLCOperandTag>');  TreatAsAtomicUnit=on
  RungOut : Outport  OutDataTypeStr=BOOL  PortDimensions=1  InitialOutput=false  VectorParamsAs1DForOutWhenUnconnected=off
  wires:
  BlockEnableRead/1(Out1) -> Instruction_Enable/Enable, __Format/1(BlockEnable)
  RungIn/1 -> RungInOverride/1(In1)
  RungInOverride/1(Out1) -> Instruction_Enable/1(Rung-condition-in), __Format/3(RungOut), __Format/2(RungIn), RungOut/1
  __CoreVarRead/1(y) -> __Format/4(data)

== system Lab2/PLC Controller Suite/__Logic/Task/Program/__Logic/OTL2 ==
  RungIn : Inport  PortDimensions=1
  BlockEnableRead : Subsystem  DisableCoverage=on  TreatAsAtomicUnit=on  mask{PLCLabelTag=_Block_Enable, PLCBlockType=BlockEnableRead}
      mask prompts: PLCLabelTag "Label Tag:"
      mask init:
      | block = gcb;
      | maskObj = Simulink.Mask.get(block);
      | maskObj.Display = sprintf('disp(''%s'');', PLCLabelTag);
      mask Help: web([docroot '/plccoder/ref/blockenableread' '.html']);
      mask DialogControl PLCBlockTitle Prompt: Block Enable Read
      mask Display: disp('_Block_Enable');
  Instruction_Enable : Subsystem  Priority=12  TreatAsAtomicUnit=on
  RungInOverride : Subsystem  DisableCoverage=on  TreatAsAtomicUnit=on
  __CoreVarRead : Subsystem  Tag=CoreVarReadBlock  DisableCoverage=on  TreatAsAtomicUnit=on  mask{PLCBlockType=CoreVarRead}
      mask init:
      | slplc.callbacks.initCoreVariable(gcb, 'read');
      mask Help: web([docroot '/plccoder/ref/__corevarread' '.html']);
      mask DialogControl PLCBlockTitle Prompt: Core Variable Read
  __Format : MATLAB Function  Tag=PLC_Format_Boolean  Priority=20  DisableCoverage=on  InitFcn=slplc.utils.setBlockAppearance('reset', '%<PLCOperandTag>');  StopFcn=slplc.utils.setBlockAppearance('reset', '%<PLCOperandTag>');  TreatAsAtomicUnit=on
  RungOut : Outport  OutDataTypeStr=BOOL  PortDimensions=1  InitialOutput=false  VectorParamsAs1DForOutWhenUnconnected=off
  wires:
  BlockEnableRead/1(Out1) -> Instruction_Enable/Enable, __Format/1(BlockEnable)
  RungIn/1 -> RungInOverride/1(In1)
  RungInOverride/1(Out1) -> Instruction_Enable/1(Rung-condition-in), __Format/3(RungOut), __Format/2(RungIn), RungOut/1
  __CoreVarRead/1(y) -> __Format/4(data)

== system Lab2/PLC Controller Suite/__Logic/Task/Program/__Logic/OTL3 ==
  RungIn : Inport  PortDimensions=1
  BlockEnableRead : Subsystem  DisableCoverage=on  TreatAsAtomicUnit=on  mask{PLCLabelTag=_Block_Enable, PLCBlockType=BlockEnableRead}
      mask prompts: PLCLabelTag "Label Tag:"
      mask init:
      | block = gcb;
      | maskObj = Simulink.Mask.get(block);
      | maskObj.Display = sprintf('disp(''%s'');', PLCLabelTag);
      mask Help: web([docroot '/plccoder/ref/blockenableread' '.html']);
      mask DialogControl PLCBlockTitle Prompt: Block Enable Read
      mask Display: disp('_Block_Enable');
  Instruction_Enable : Subsystem  Priority=12  TreatAsAtomicUnit=on
  RungInOverride : Subsystem  DisableCoverage=on  TreatAsAtomicUnit=on
  __CoreVarRead : Subsystem  Tag=CoreVarReadBlock  DisableCoverage=on  TreatAsAtomicUnit=on  mask{PLCBlockType=CoreVarRead}
      mask init:
      | slplc.callbacks.initCoreVariable(gcb, 'read');
      mask Help: web([docroot '/plccoder/ref/__corevarread' '.html']);
      mask DialogControl PLCBlockTitle Prompt: Core Variable Read
  __Format : MATLAB Function  Tag=PLC_Format_Boolean  Priority=20  DisableCoverage=on  InitFcn=slplc.utils.setBlockAppearance('reset', '%<PLCOperandTag>');  StopFcn=slplc.utils.setBlockAppearance('reset', '%<PLCOperandTag>');  TreatAsAtomicUnit=on
  RungOut : Outport  OutDataTypeStr=BOOL  PortDimensions=1  InitialOutput=false  VectorParamsAs1DForOutWhenUnconnected=off
  wires:
  BlockEnableRead/1(Out1) -> Instruction_Enable/Enable, __Format/1(BlockEnable)
  RungIn/1 -> RungInOverride/1(In1)
  RungInOverride/1(Out1) -> Instruction_Enable/1(Rung-condition-in), __Format/3(RungOut), __Format/2(RungIn), RungOut/1
  __CoreVarRead/1(y) -> __Format/4(data)

== system Lab2/PLC Controller Suite/__Logic/Task/Program/__Logic/OTL4 ==
  RungIn : Inport  PortDimensions=1
  BlockEnableRead : Subsystem  DisableCoverage=on  TreatAsAtomicUnit=on  mask{PLCLabelTag=_Block_Enable, PLCBlockType=BlockEnableRead}
      mask prompts: PLCLabelTag "Label Tag:"
      mask init:
      | block = gcb;
      | maskObj = Simulink.Mask.get(block);
      | maskObj.Display = sprintf('disp(''%s'');', PLCLabelTag);
      mask Help: web([docroot '/plccoder/ref/blockenableread' '.html']);
      mask DialogControl PLCBlockTitle Prompt: Block Enable Read
      mask Display: disp('_Block_Enable');
  Instruction_Enable : Subsystem  Priority=12  TreatAsAtomicUnit=on
  RungInOverride : Subsystem  DisableCoverage=on  TreatAsAtomicUnit=on
  __CoreVarRead : Subsystem  Tag=CoreVarReadBlock  DisableCoverage=on  TreatAsAtomicUnit=on  mask{PLCBlockType=CoreVarRead}
      mask init:
      | slplc.callbacks.initCoreVariable(gcb, 'read');
      mask Help: web([docroot '/plccoder/ref/__corevarread' '.html']);
      mask DialogControl PLCBlockTitle Prompt: Core Variable Read
  __Format : MATLAB Function  Tag=PLC_Format_Boolean  Priority=20  DisableCoverage=on  InitFcn=slplc.utils.setBlockAppearance('reset', '%<PLCOperandTag>');  StopFcn=slplc.utils.setBlockAppearance('reset', '%<PLCOperandTag>');  TreatAsAtomicUnit=on
  RungOut : Outport  OutDataTypeStr=BOOL  PortDimensions=1  InitialOutput=false  VectorParamsAs1DForOutWhenUnconnected=off
  wires:
  BlockEnableRead/1(Out1) -> Instruction_Enable/Enable, __Format/1(BlockEnable)
  RungIn/1 -> RungInOverride/1(In1)
  RungInOverride/1(Out1) -> Instruction_Enable/1(Rung-condition-in), __Format/3(RungOut), __Format/2(RungIn), RungOut/1
  __CoreVarRead/1(y) -> __Format/4(data)

== system Lab2/PLC Controller Suite/__Logic/Task/Program/__Logic/OTU ==
  RungIn : Inport  PortDimensions=1
  BlockEnableRead : Subsystem  DisableCoverage=on  TreatAsAtomicUnit=on  mask{PLCLabelTag=_Block_Enable, PLCBlockType=BlockEnableRead}
      mask prompts: PLCLabelTag "Label Tag:"
      mask init:
      | block = gcb;
      | maskObj = Simulink.Mask.get(block);
      | maskObj.Display = sprintf('disp(''%s'');', PLCLabelTag);
      mask Help: web([docroot '/plccoder/ref/blockenableread' '.html']);
      mask DialogControl PLCBlockTitle Prompt: Block Enable Read
      mask Display: disp('_Block_Enable');
  Instruction_Enable : Subsystem  Priority=12  TreatAsAtomicUnit=on
  RungInOverride : Subsystem  DisableCoverage=on  TreatAsAtomicUnit=on
  __CoreVarRead : Subsystem  Tag=CoreVarReadBlock  DisableCoverage=on  TreatAsAtomicUnit=on  mask{PLCBlockType=CoreVarRead}
      mask init:
      | slplc.callbacks.initCoreVariable(gcb, 'read');
      mask Help: web([docroot '/plccoder/ref/__corevarread' '.html']);
      mask DialogControl PLCBlockTitle Prompt: Core Variable Read
  __Format : MATLAB Function  Tag=PLC_Format_Boolean  Priority=20  DisableCoverage=on  InitFcn=slplc.utils.setBlockAppearance('reset', '%<PLCOperandTag>');  StopFcn=slplc.utils.setBlockAppearance('reset', '%<PLCOperandTag>');  TreatAsAtomicUnit=on
  RungOut : Outport  OutDataTypeStr=BOOL  PortDimensions=1  InitialOutput=false  VectorParamsAs1DForOutWhenUnconnected=off
  wires:
  RungIn/1 -> RungInOverride/1(In1)
  RungInOverride/1(Out1) -> __Format/3(RungOut), __Format/2(RungIn), RungOut/1, Instruction_Enable/1(Rung-condition-in)
  BlockEnableRead/1(Out1) -> Instruction_Enable/Enable, __Format/1(BlockEnable)
  __CoreVarRead/1(y) -> __Format/4(data)

== system Lab2/PLC Controller Suite/__Logic/Task/Program/__Logic/OTU1 ==
  RungIn : Inport  PortDimensions=1
  BlockEnableRead : Subsystem  DisableCoverage=on  TreatAsAtomicUnit=on  mask{PLCLabelTag=_Block_Enable, PLCBlockType=BlockEnableRead}
      mask prompts: PLCLabelTag "Label Tag:"
      mask init:
      | block = gcb;
      | maskObj = Simulink.Mask.get(block);
      | maskObj.Display = sprintf('disp(''%s'');', PLCLabelTag);
      mask Help: web([docroot '/plccoder/ref/blockenableread' '.html']);
      mask DialogControl PLCBlockTitle Prompt: Block Enable Read
      mask Display: disp('_Block_Enable');
  Instruction_Enable : Subsystem  Priority=12  TreatAsAtomicUnit=on
  RungInOverride : Subsystem  DisableCoverage=on  TreatAsAtomicUnit=on
  __CoreVarRead : Subsystem  Tag=CoreVarReadBlock  DisableCoverage=on  TreatAsAtomicUnit=on  mask{PLCBlockType=CoreVarRead}
      mask init:
      | slplc.callbacks.initCoreVariable(gcb, 'read');
      mask Help: web([docroot '/plccoder/ref/__corevarread' '.html']);
      mask DialogControl PLCBlockTitle Prompt: Core Variable Read
  __Format : MATLAB Function  Tag=PLC_Format_Boolean  Priority=20  DisableCoverage=on  InitFcn=slplc.utils.setBlockAppearance('reset', '%<PLCOperandTag>');  StopFcn=slplc.utils.setBlockAppearance('reset', '%<PLCOperandTag>');  TreatAsAtomicUnit=on
  RungOut : Outport  OutDataTypeStr=BOOL  PortDimensions=1  InitialOutput=false  VectorParamsAs1DForOutWhenUnconnected=off
  wires:
  RungIn/1 -> RungInOverride/1(In1)
  RungInOverride/1(Out1) -> __Format/3(RungOut), __Format/2(RungIn), RungOut/1, Instruction_Enable/1(Rung-condition-in)
  BlockEnableRead/1(Out1) -> Instruction_Enable/Enable, __Format/1(BlockEnable)
  __CoreVarRead/1(y) -> __Format/4(data)

== system Lab2/PLC Controller Suite/__Logic/Task/Program/__Logic/Power Rail Start ==
  PLCPowerOn : Constant  Value=true  OutDataTypeStr=BOOL
  __Format : MATLAB Function  Tag=PLC_Format_ENO  Priority=20  DisableCoverage=on  InitFcn=slplc.utils.setBlockAppearance('reset', '', {'black', 'black'});  StopFcn=slplc.utils.setBlockAppearance('reset', '', {'black', 'black'});  TreatAsAtomicUnit=on
  PowerOut : Outport  VectorParamsAs1DForOutWhenUnconnected=off
  wires:
  PLCPowerOn/1 -> __Format/1(RungOut), PowerOut/1

== system Lab2/PLC Controller Suite/__Logic/Task/Program/__Logic/Power Rail Terminal ==
  PowerIn : Inport
  Terminator3 : Terminator
  wires:
  PowerIn/1 -> Terminator3/1

== system Lab2/PLC Controller Suite/__Logic/Task/Program/__Logic/Program Variables ==

== system Lab2/PLC Controller Suite/__Logic/Task/Program/__Logic/Rung Terminal ==
  RungIn : Inport
  Terminator : Terminator
  wires:
  RungIn/1 -> Terminator/1

== system Lab2/PLC Controller Suite/__Logic/Task/Program/__Logic/Rung Terminal1 ==
  RungIn : Inport
  Terminator : Terminator
  wires:
  RungIn/1 -> Terminator/1

== system Lab2/PLC Controller Suite/__Logic/Task/Program/__Logic/Rung Terminal2 ==
  RungIn : Inport
  Terminator : Terminator
  wires:
  RungIn/1 -> Terminator/1

== system Lab2/PLC Controller Suite/__Logic/Task/Program/__Logic/Rung Terminal3 ==
  RungIn : Inport
  Terminator : Terminator
  wires:
  RungIn/1 -> Terminator/1

== system Lab2/PLC Controller Suite/__Logic/Task/Program/__Logic/Up to Parent POU ==

== system Lab2/PLC Controller Suite/__Logic/Task/Program/__Logic/Variable Read ==
  __CoreVarRead : Subsystem  Tag=CoreVarReadBlock  DisableCoverage=on  TreatAsAtomicUnit=on  mask{PLCBlockType=CoreVarRead}
      mask init:
      | slplc.callbacks.initCoreVariable(gcb, 'read');
      mask Help: web([docroot '/plccoder/ref/__corevarread' '.html']);
      mask DialogControl PLCBlockTitle Prompt: Core Variable Read
  __Format : MATLAB Function  Tag=PLC_Format_Data  Priority=20  DisableCoverage=on  InitFcn=slplc.utils.setBlockAppearance('reset');  StopFcn=slplc.utils.setBlockAppearance('reset');  TreatAsAtomicUnit=on
  VarOut : Outport  VectorParamsAs1DForOutWhenUnconnected=off
  wires:
  __CoreVarRead/1(y) -> __Format/1(data), VarOut/1
